simulink model "airTrackLab"  (R2021a)
settings: Solver=ode23t  StartTime=0.0  StopTime=30  FixedStep=0.02  MaxStep=0.01  RelTol=1e-3  AbsTol=1e-4  EnableMultiTasking=on
PostLoadFcn:
  | disp('default settings')
  | 
  | % Default starting positions
  | x0_cart1 = -0.2
  | x0_cart2 = 0.8
  | x0_gate1 = -0.4
  | x0_gate2 = 0.4
  | 
  | % How much damping the carts feel
  | dampingCoef = 0.01 % N/(m/s)
  | 
  | % Hanger damping
  | pulleyDamping = 0;
  | 
  | % Max measurement noise for the gates
  | noise_max = 0.01 % seconds
  | 
  | % How many time steps to show in the history
  | nHistory = 4
  | 
  | % Based on the provided STLs
  | cart_length = 0.15
  | 
  | subsystems = find_system(gcs,'BlockType','SubSystem');
  | p = Simulink.Mask.get(subsystems{1});
  | p.Parameters(1).Value = '-0.8';
  | p.Parameters(2).Value = '0';
  | p.Parameters(3).Value = '-0.4';
  | p.Parameters(4).Value = '0.4';
  | p.Parameters(5).Value = '0';
  | p.Parameters(6).Value = '0';
  | 
  | % Resize the model window
  | set(0,"Units","pixels")
  | sSize = get(0,"screensize");
  | set_param(gcs,'location',...
  |     [1,sSize(4)*0.01,round(sSize(3)/2),sSize(4)*0.96]);
  | 
  | % Reset the zoom
  | set_param(gcs, 'ZoomFactor','FitSystem')
undefined symbols (not defined in the file): X, Y, Z
libraries: sm_lib x104, simulink x12, nesl_utility x9
(part 3 of 3)

== system airTrackLab/Air track model/Mass Cart 1/Plates 3 ==
  Plate 1 : sm_lib/Body Elements/File Solid  ExtGeomFileName=weight.stl  UnitType=Custom  ExtGeomFileUnits=mm  StepReaderType=HEX  ExportConvexHullGeometry=off  InertiaType=PointMass  Mass=100  MassUnits=g  CenterOfMass=[0 0 0]  CenterOfMassUnits=m  MomentsOfInertia=[1 1 1]  MomentsOfInertiaUnits=kg*m^2  ProductsOfInertia=[0 0 0]  ProductsOfInertiaUnits=kg*m^2  BasedOnType=Density  Density=1000  DensityUnits=kg/m^3  DoExposeReferenceFrame=on  SerializedFrames=<Frames/>  GraphicType=FromGeometry  MarkerShape=Sphere  MarkerSize=10  GraphicVisPropType=AdvancedVisualProperties  GraphicDiffuseColor="[0.70   0.7    0.3]"  GraphicSpecularColor="[0.7  0.7  0.5 1]"  GraphicAmbientColor=[0.05 0.05 0.05 1]  GraphicEmissiveColor=[0.2 0.2 0.2 1.0]  GraphicShininess=3  GraphicOpacity=1.0
  Plate 2 : sm_lib/Body Elements/File Solid  ExtGeomFileName=weight.stl  UnitType=Custom  ExtGeomFileUnits=mm  StepReaderType=HEX  ExportConvexHullGeometry=off  InertiaType=PointMass  Mass=100  MassUnits=g  CenterOfMass=[0 0 0]  CenterOfMassUnits=m  MomentsOfInertia=[1 1 1]  MomentsOfInertiaUnits=kg*m^2  ProductsOfInertia=[0 0 0]  ProductsOfInertiaUnits=kg*m^2  BasedOnType=Density  Density=1000  DensityUnits=kg/m^3  DoExposeReferenceFrame=on  SerializedFrames=<Frames/>  GraphicType=FromGeometry  MarkerShape=Sphere  MarkerSize=10  GraphicVisPropType=AdvancedVisualProperties  GraphicDiffuseColor="[0.70   0.7    0.3]"  GraphicSpecularColor="[0.7  0.7  0.5 1]"  GraphicAmbientColor=[0.05 0.05 0.05 1]  GraphicEmissiveColor=[0.2 0.2 0.2 1.0]  GraphicShininess=3  GraphicOpacity=1.0
  Plate 3 : sm_lib/Body Elements/File Solid  ExtGeomFileName=weight.stl  UnitType=Custom  ExtGeomFileUnits=mm  StepReaderType=HEX  ExportConvexHullGeometry=off  InertiaType=PointMass  Mass=100  MassUnits=g  CenterOfMass=[0 0 0]  CenterOfMassUnits=m  MomentsOfInertia=[1 1 1]  MomentsOfInertiaUnits=kg*m^2  ProductsOfInertia=[0 0 0]  ProductsOfInertiaUnits=kg*m^2  BasedOnType=Density  Density=1000  DensityUnits=kg/m^3  DoExposeReferenceFrame=on  SerializedFrames=<Frames/>  GraphicType=FromGeometry  MarkerShape=Sphere  MarkerSize=10  GraphicVisPropType=AdvancedVisualProperties  GraphicDiffuseColor="[0.70   0.7    0.3]"  GraphicSpecularColor="[0.7  0.7  0.5 1]"  GraphicAmbientColor=[0.05 0.05 0.05 1]  GraphicEmissiveColor=[0.2 0.2 0.2 1.0]  GraphicShininess=3  GraphicOpacity=1.0
  Transform Plate 1 : sm_lib/Frames and Transforms/Rigid Transform  TranslationMethod=Cartesian  TranslationStandardOffset=0  TranslationLengthUnit=m  TranslationStandardAxis=+Z  TranslationCartesianOffset=[0 0.0055 0.0]  TranslationROffset=0  TranslationROffsetUnits=m  TranslationZOffset=0  TranslationZOffsetUnits=m  TranslationThetaOffset=0  TranslationThetaOffsetUnits=deg  RotationMethod=None  RotationAngleUnits=deg  RotationStandardAxis=+Z  RotationAngle=0.0  RotationArbitraryAxis=[0 0 1]  FollAlignAxisA=+X  BaseAlignAxisA=+Y  FollAlignAxisB=+Y  BaseAlignAxisB=+Z  RotationSequenceAxes=FollowerAxes  RotationSequence=XYX  RotationSequenceAngles=[0 0 0]  RotationSequenceAnglesUnits=deg  RotationMatrix=[1 0 0; 0 1 0; 0 0 1]
  Transform Plate 2 : sm_lib/Frames and Transforms/Rigid Transform  TranslationMethod=Cartesian  TranslationStandardOffset=0  TranslationLengthUnit=m  TranslationStandardAxis=+Z  TranslationCartesianOffset=[0 0.0055 0.0]  TranslationROffset=0  TranslationROffsetUnits=m  TranslationZOffset=0  TranslationZOffsetUnits=m  TranslationThetaOffset=0  TranslationThetaOffsetUnits=deg  RotationMethod=None  RotationAngleUnits=deg  RotationStandardAxis=+Z  RotationAngle=0.0  RotationArbitraryAxis=[0 0 1]  FollAlignAxisA=+X  BaseAlignAxisA=+Y  FollAlignAxisB=+Y  BaseAlignAxisB=+Z  RotationSequenceAxes=FollowerAxes  RotationSequence=XYX  RotationSequenceAngles=[0 0 0]  RotationSequenceAnglesUnits=deg  RotationMatrix=[1 0 0; 0 1 0; 0 0 1]
  Transform Plate 3 : sm_lib/Frames and Transforms/Rigid Transform  TranslationMethod=Cartesian  TranslationStandardOffset=0  TranslationLengthUnit=m  TranslationStandardAxis=+Z  TranslationCartesianOffset=[0 0.0055 0.0]  TranslationROffset=0  TranslationROffsetUnits=m  TranslationZOffset=0  TranslationZOffsetUnits=m  TranslationThetaOffset=0  TranslationThetaOffsetUnits=deg  RotationMethod=None  RotationAngleUnits=deg  RotationStandardAxis=+Z  RotationAngle=0.0  RotationArbitraryAxis=[0 0 1]  FollAlignAxisA=+X  BaseAlignAxisA=+Y  FollAlignAxisB=+Y  BaseAlignAxisB=+Z  RotationSequenceAxes=FollowerAxes  RotationSequence=XYX  RotationSequenceAngles=[0 0 0]  RotationSequenceAnglesUnits=deg  RotationMatrix=[1 0 0; 0 1 0; 0 0 1]
  B : PMIOPort  Side=Right
  connections:
  Plate 2/RConn1 -- Transform Plate 2/RConn1 -- Transform Plate 3/LConn1
  Transform Plate 1/LConn1 -- B/RConn1
  Transform Plate 2/LConn1 -- Plate 1/RConn1 -- Transform Plate 1/RConn1
  Plate 3/RConn1 -- Transform Plate 3/RConn1

== system airTrackLab/Air track model/Mass Cart 2/None  ==
  Reference Frame : sm_lib/Frames and Transforms/Reference Frame
  B : PMIOPort  Side=Right
  connections:
  B/RConn1 -- Reference Frame/RConn1

== system airTrackLab/Air track model/Mass Cart 2/Plates 1 ==
  Plate 1 : sm_lib/Body Elements/File Solid  ExtGeomFileName=weight.stl  UnitType=Custom  ExtGeomFileUnits=mm  StepReaderType=HEX  ExportConvexHullGeometry=off  InertiaType=PointMass  Mass=100  MassUnits=g  CenterOfMass=[0 0 0]  CenterOfMassUnits=m  MomentsOfInertia=[1 1 1]  MomentsOfInertiaUnits=kg*m^2  ProductsOfInertia=[0 0 0]  ProductsOfInertiaUnits=kg*m^2  BasedOnType=Density  Density=1000  DensityUnits=kg/m^3  DoExposeReferenceFrame=on  SerializedFrames=<Frames/>  GraphicType=FromGeometry  MarkerShape=Sphere  MarkerSize=10  GraphicVisPropType=AdvancedVisualProperties  GraphicDiffuseColor="[0.70   0.7    0.3]"  GraphicSpecularColor="[0.7  0.7  0.5 1]"  GraphicAmbientColor=[0.05 0.05 0.05 1]  GraphicEmissiveColor=[0.2 0.2 0.2 1.0]  GraphicShininess=3  GraphicOpacity=1.0
  Transform Plate 1 : sm_lib/Frames and Transforms/Rigid Transform  TranslationMethod=Cartesian  TranslationStandardOffset=0  TranslationLengthUnit=m  TranslationStandardAxis=+Z  TranslationCartesianOffset=[0 0.0055 0.0]  TranslationROffset=0  TranslationROffsetUnits=m  TranslationZOffset=0  TranslationZOffsetUnits=m  TranslationThetaOffset=0  TranslationThetaOffsetUnits=deg  RotationMethod=None  RotationAngleUnits=deg  RotationStandardAxis=+Z  RotationAngle=0.0  RotationArbitraryAxis=[0 0 1]  FollAlignAxisA=+X  BaseAlignAxisA=+Y  FollAlignAxisB=+Y  BaseAlignAxisB=+Z  RotationSequenceAxes=FollowerAxes  RotationSequence=XYX  RotationSequenceAngles=[0 0 0]  RotationSequenceAnglesUnits=deg  RotationMatrix=[1 0 0; 0 1 0; 0 0 1]
  B : PMIOPort  Side=Right
  connections:
  Plate 1/RConn1 -- Transform Plate 1/RConn1
  Transform Plate 1/LConn1 -- B/RConn1

== system airTrackLab/Air track model/Mass Cart 2/Plates 2 ==
  Plate 1 : sm_lib/Body Elements/File Solid  ExtGeomFileName=weight.stl  UnitType=Custom  ExtGeomFileUnits=mm  StepReaderType=HEX  ExportConvexHullGeometry=off  InertiaType=PointMass  Mass=100  MassUnits=g  CenterOfMass=[0 0 0]  CenterOfMassUnits=m  MomentsOfInertia=[1 1 1]  MomentsOfInertiaUnits=kg*m^2  ProductsOfInertia=[0 0 0]  ProductsOfInertiaUnits=kg*m^2  BasedOnType=Density  Density=1000  DensityUnits=kg/m^3  DoExposeReferenceFrame=on  SerializedFrames=<Frames/>  GraphicType=FromGeometry  MarkerShape=Sphere  MarkerSize=10  GraphicVisPropType=AdvancedVisualProperties  GraphicDiffuseColor="[0.70   0.7    0.3]"  GraphicSpecularColor="[0.7  0.7  0.5 1]"  GraphicAmbientColor=[0.05 0.05 0.05 1]  GraphicEmissiveColor=[0.2 0.2 0.2 1.0]  GraphicShininess=3  GraphicOpacity=1.0
  Plate 2 : sm_lib/Body Elements/File Solid  ExtGeomFileName=weight.stl  UnitType=Custom  ExtGeomFileUnits=mm  StepReaderType=HEX  ExportConvexHullGeometry=off  InertiaType=PointMass  Mass=100  MassUnits=g  CenterOfMass=[0 0 0]  CenterOfMassUnits=m  MomentsOfInertia=[1 1 1]  MomentsOfInertiaUnits=kg*m^2  ProductsOfInertia=[0 0 0]  ProductsOfInertiaUnits=kg*m^2  BasedOnType=Density  Density=1000  DensityUnits=kg/m^3  DoExposeReferenceFrame=on  SerializedFrames=<Frames/>  GraphicType=FromGeometry  MarkerShape=Sphere  MarkerSize=10  GraphicVisPropType=AdvancedVisualProperties  GraphicDiffuseColor="[0.70   0.7    0.3]"  GraphicSpecularColor="[0.7  0.7  0.5 1]"  GraphicAmbientColor=[0.05 0.05 0.05 1]  GraphicEmissiveColor=[0.2 0.2 0.2 1.0]  GraphicShininess=3  GraphicOpacity=1.0
  Transform Plate 1 : sm_lib/Frames and Transforms/Rigid Transform  TranslationMethod=Cartesian  TranslationStandardOffset=0  TranslationLengthUnit=m  TranslationStandardAxis=+Z  TranslationCartesianOffset=[0 0.0055 0.0]  TranslationROffset=0  TranslationROffsetUnits=m  TranslationZOffset=0  TranslationZOffsetUnits=m  TranslationThetaOffset=0  TranslationThetaOffsetUnits=deg  RotationMethod=None  RotationAngleUnits=deg  RotationStandardAxis=+Z  RotationAngle=0.0  RotationArbitraryAxis=[0 0 1]  FollAlignAxisA=+X  BaseAlignAxisA=+Y  FollAlignAxisB=+Y  BaseAlignAxisB=+Z  RotationSequenceAxes=FollowerAxes  RotationSequence=XYX  RotationSequenceAngles=[0 0 0]  RotationSequenceAnglesUnits=deg  RotationMatrix=[1 0 0; 0 1 0; 0 0 1]
  Transform Plate 2 : sm_lib/Frames and Transforms/Rigid Transform  TranslationMethod=Cartesian  TranslationStandardOffset=0  TranslationLengthUnit=m  TranslationStandardAxis=+Z  TranslationCartesianOffset=[0 0.0055 0.0]  TranslationROffset=0  TranslationROffsetUnits=m  TranslationZOffset=0  TranslationZOffsetUnits=m  TranslationThetaOffset=0  TranslationThetaOffsetUnits=deg  RotationMethod=None  RotationAngleUnits=deg  RotationStandardAxis=+Z  RotationAngle=0.0  RotationArbitraryAxis=[0 0 1]  FollAlignAxisA=+X  BaseAlignAxisA=+Y  FollAlignAxisB=+Y  BaseAlignAxisB=+Z  RotationSequenceAxes=FollowerAxes  RotationSequence=XYX  RotationSequenceAngles=[0 0 0]  RotationSequenceAnglesUnits=deg  RotationMatrix=[1 0 0; 0 1 0; 0 0 1]
  B : PMIOPort  Side=Right
  connections:
  Plate 2/RConn1 -- Transform Plate 2/RConn1
  Transform Plate 1/LConn1 -- B/RConn1
  Transform Plate 1/RConn1 -- Transform Plate 2/LConn1 -- Plate 1/RConn1

== system airTrackLab/Air track model/Mass Cart 2/Plates 3 ==
  Plate 1 : sm_lib/Body Elements/File Solid  ExtGeomFileName=weight.stl  UnitType=Custom  ExtGeomFileUnits=mm  StepReaderType=HEX  ExportConvexHullGeometry=off  InertiaType=PointMass  Mass=100  MassUnits=g  CenterOfMass=[0 0 0]  CenterOfMassUnits=m  MomentsOfInertia=[1 1 1]  MomentsOfInertiaUnits=kg*m^2  ProductsOfInertia=[0 0 0]  ProductsOfInertiaUnits=kg*m^2  BasedOnType=Density  Density=1000  DensityUnits=kg/m^3  DoExposeReferenceFrame=on  SerializedFrames=<Frames/>  GraphicType=FromGeometry  MarkerShape=Sphere  MarkerSize=10  GraphicVisPropType=AdvancedVisualProperties  GraphicDiffuseColor="[0.70   0.7    0.3]"  GraphicSpecularColor="[0.7  0.7  0.5 1]"  GraphicAmbientColor=[0.05 0.05 0.05 1]  GraphicEmissiveColor=[0.2 0.2 0.2 1.0]  GraphicShininess=3  GraphicOpacity=1.0
  Plate 2 : sm_lib/Body Elements/File Solid  ExtGeomFileName=weight.stl  UnitType=Custom  ExtGeomFileUnits=mm  StepReaderType=HEX  ExportConvexHullGeometry=off  InertiaType=PointMass  Mass=100  MassUnits=g  CenterOfMass=[0 0 0]  CenterOfMassUnits=m  MomentsOfInertia=[1 1 1]  MomentsOfInertiaUnits=kg*m^2  ProductsOfInertia=[0 0 0]  ProductsOfInertiaUnits=kg*m^2  BasedOnType=Density  Density=1000  DensityUnits=kg/m^3  DoExposeReferenceFrame=on  SerializedFrames=<Frames/>  GraphicType=FromGeometry  MarkerShape=Sphere  MarkerSize=10  GraphicVisPropType=AdvancedVisualProperties  GraphicDiffuseColor="[0.70   0.7    0.3]"  GraphicSpecularColor="[0.7  0.7  0.5 1]"  GraphicAmbientColor=[0.05 0.05 0.05 1]  GraphicEmissiveColor=[0.2 0.2 0.2 1.0]  GraphicShininess=3  GraphicOpacity=1.0
  Plate 3 : sm_lib/Body Elements/File Solid  ExtGeomFileName=weight.stl  UnitType=Custom  ExtGeomFileUnits=mm  StepReaderType=HEX  ExportConvexHullGeometry=off  InertiaType=PointMass  Mass=100  MassUnits=g  CenterOfMass=[0 0 0]  CenterOfMassUnits=m  MomentsOfInertia=[1 1 1]  MomentsOfInertiaUnits=kg*m^2  ProductsOfInertia=[0 0 0]  ProductsOfInertiaUnits=kg*m^2  BasedOnType=Density  Density=1000  DensityUnits=kg/m^3  DoExposeReferenceFrame=on  SerializedFrames=<Frames/>  GraphicType=FromGeometry  MarkerShape=Sphere  MarkerSize=10  GraphicVisPropType=AdvancedVisualProperties  GraphicDiffuseColor="[0.70   0.7    0.3]"  GraphicSpecularColor="[0.7  0.7  0.5 1]"  GraphicAmbientColor=[0.05 0.05 0.05 1]  GraphicEmissiveColor=[0.2 0.2 0.2 1.0]  GraphicShininess=3  GraphicOpacity=1.0
  Transform Plate 1 : sm_lib/Frames and Transforms/Rigid Transform  TranslationMethod=Cartesian  TranslationStandardOffset=0  TranslationLengthUnit=m  TranslationStandardAxis=+Z  TranslationCartesianOffset=[0 0.0055 0.0]  TranslationROffset=0  TranslationROffsetUnits=m  TranslationZOffset=0  TranslationZOffsetUnits=m  TranslationThetaOffset=0  TranslationThetaOffsetUnits=deg  RotationMethod=None  RotationAngleUnits=deg  RotationStandardAxis=+Z  RotationAngle=0.0  RotationArbitraryAxis=[0 0 1]  FollAlignAxisA=+X  BaseAlignAxisA=+Y  FollAlignAxisB=+Y  BaseAlignAxisB=+Z  RotationSequenceAxes=FollowerAxes  RotationSequence=XYX  RotationSequenceAngles=[0 0 0]  RotationSequenceAnglesUnits=deg  RotationMatrix=[1 0 0; 0 1 0; 0 0 1]
  Transform Plate 2 : sm_lib/Frames and Transforms/Rigid Transform  TranslationMethod=Cartesian  TranslationStandardOffset=0  TranslationLengthUnit=m  TranslationStandardAxis=+Z  TranslationCartesianOffset=[0 0.0055 0.0]  TranslationROffset=0  TranslationROffsetUnits=m  TranslationZOffset=0  TranslationZOffsetUnits=m  TranslationThetaOffset=0  TranslationThetaOffsetUnits=deg  RotationMethod=None  RotationAngleUnits=deg  RotationStandardAxis=+Z  RotationAngle=0.0  RotationArbitraryAxis=[0 0 1]  FollAlignAxisA=+X  BaseAlignAxisA=+Y  FollAlignAxisB=+Y  BaseAlignAxisB=+Z  RotationSequenceAxes=FollowerAxes  RotationSequence=XYX  RotationSequenceAngles=[0 0 0]  RotationSequenceAnglesUnits=deg  RotationMatrix=[1 0 0; 0 1 0; 0 0 1]
  Transform Plate 3 : sm_lib/Frames and Transforms/Rigid Transform  TranslationMethod=Cartesian  TranslationStandardOffset=0  TranslationLengthUnit=m  TranslationStandardAxis=+Z  TranslationCartesianOffset=[0 0.0055 0.0]  TranslationROffset=0  TranslationROffsetUnits=m  TranslationZOffset=0  TranslationZOffsetUnits=m  TranslationThetaOffset=0  TranslationThetaOffsetUnits=deg  RotationMethod=None  RotationAngleUnits=deg  RotationStandardAxis=+Z  RotationAngle=0.0  RotationArbitraryAxis=[0 0 1]  FollAlignAxisA=+X  BaseAlignAxisA=+Y  FollAlignAxisB=+Y  BaseAlignAxisB=+Z  RotationSequenceAxes=FollowerAxes  RotationSequence=XYX  RotationSequenceAngles=[0 0 0]  RotationSequenceAnglesUnits=deg  RotationMatrix=[1 0 0; 0 1 0; 0 0 1]
  B : PMIOPort  Side=Right
  connections:
  Plate 3/RConn1 -- Transform Plate 3/RConn1
  Transform Plate 1/RConn1 -- Plate 1/RConn1 -- Transform Plate 2/LConn1
  Transform Plate 1/LConn1 -- B/RConn1
  Transform Plate 3/LConn1 -- Transform Plate 2/RConn1 -- Plate 2/RConn1

== system airTrackLab/Air track model/Force Cart 1/short pulse/Triggered Subsystem ==
  In1 : Inport
  Trigger : TriggerPort  VariantControl=Variant
  Out1 : Outport
  wires:
  In1/1 -> Out1/1

== system airTrackLab/Air track model/Force Cart 1/short pulse/Triggered Subsystem1 ==
  In1 : Inport
  Trigger : TriggerPort  VariantControl=Variant
  Out1 : Outport
  wires:
  In1/1 -> Out1/1

== system airTrackLab/Air track model/Force Cart 2/Interactive Pulse/Triggered Subsystem ==
  In1 : Inport
  Trigger : TriggerPort  VariantControl=Variant
  Out1 : Outport
  wires:
  In1/1 -> Out1/1

== system airTrackLab/Air track model/Force Cart 2/Interactive Pulse/Triggered Subsystem1 ==
  In1 : Inport
  Trigger : TriggerPort  VariantControl=Variant
  Out1 : Outport
  wires:
  In1/1 -> Out1/1

== system airTrackLab/Air track model/Gate 1/Gate timing and history/Gate Trigger1 ==
  note: If the cart passes close to the gate, take a recording
      | (only triggers once when it comes into range)
  position1 : Inport
  velocity1 : Inport  Port=2
  gate_pos : Inport  Port=3
  Abs : Abs
  Compare To Constant : simulink/Logic and Bit Operations/Compare To Constant  relop=<=  const=0.01  OutDataTypeStr=boolean
  Subtract : Sum  Inputs=+-
  Uniform Random Number1 : UniformRandomNumber  Minimum=-noise_max/2  Maximum=noise_max/2  SampleTime=0.1
  gate 1 recording : Subsystem  TreatAsAtomicUnit=on
  cart time : Outport
  wires:
  position1/1 -> Subtract/2
  velocity1/1 -> gate 1 recording/1(In1)
  gate 1 recording/1(cart time) -> cart time/1
  Abs/1 -> Compare To Constant/1
  Subtract/1 -> Abs/1
  Compare To Constant/1 -> gate 1 recording/Trigger
  Uniform Random Number1/1 -> gate 1 recording/2(In2)
  gate_pos/1 -> Subtract/1

== system airTrackLab/Air track model/Gate 1/Gate timing and history/Gate Trigger2 ==
  note: If the cart passes close to the gate, take a recording
      | (only triggers once when it comes into range)
  position1 : Inport
  velocity1 : Inport  Port=2
  gate_pos : Inport  Port=3
  Abs : Abs
  Compare To Constant : simulink/Logic and Bit Operations/Compare To Constant  relop=<=  const=0.01  OutDataTypeStr=boolean
  Subtract : Sum  Inputs=+-
  Uniform Random Number : UniformRandomNumber  Minimum=-noise_max/2  Maximum=noise_max/2  SampleTime=0.1
  gate 1 recording : Subsystem  TreatAsAtomicUnit=on
  cart time : Outport
  wires:
  position1/1 -> Subtract/2
  velocity1/1 -> gate 1 recording/1(In1)
  gate 1 recording/1(cart time) -> cart time/1
  Abs/1 -> Compare To Constant/1
  Subtract/1 -> Abs/1
  Compare To Constant/1 -> gate 1 recording/Trigger
  Uniform Random Number/1 -> gate 1 recording/2(In2)
  gate_pos/1 -> Subtract/1

== system airTrackLab/Air track model/Gate 1/Gate timing and history/Memory system ==
  value : Inport
  Assignment : Assignment  DiagnosticForDimensions=Warning  IndexOptions=Index vector (dialog)  Indices=1  OutputSizes=1
  Equal : RelationalOperator  Operator=~=  OutDataTypeStr=boolean  RndMeth=Simplest
  Triggered Subsystem : Subsystem  TreatAsAtomicUnit=on
  Unit Delay : UnitDelay  InitialCondition=zeros(nHistory,1)  SampleTime=-1  HasFrameUpgradeWarning=on
  Unit Delay1 : UnitDelay  SampleTime=-1  HasFrameUpgradeWarning=on
  last n values : Outport
  wires:
  Unit Delay/1 -> Triggered Subsystem/1(In1)
  Assignment/1 -> Unit Delay/1, last n values/1
  value/1 -> Equal/1, Unit Delay1/1, Assignment/2
  Triggered Subsystem/1(Out1) -> Assignment/1
  Equal/1 -> Triggered Subsystem/Trigger
  Unit Delay1/1 -> Equal/2

== system airTrackLab/Air track model/Gate 1/Gate timing and history/Triggered Subsystem ==
  time : Inport
  Trigger : TriggerPort  VariantControl=Variant
  timeOut : Outport
  wires:
  time/1 -> timeOut/1

== system airTrackLab/Air track model/Gate 2/Gate timing and history/Gate Trigger1 ==
  note: If the cart passes close to the gate, take a recording
      | (only triggers once when it comes into range)
  position1 : Inport
  velocity1 : Inport  Port=2
  gate_pos : Inport  Port=3
  Abs : Abs
  Compare To Constant : simulink/Logic and Bit Operations/Compare To Constant  relop=<=  const=0.01  OutDataTypeStr=boolean
  Subtract : Sum  Inputs=+-
  Uniform Random Number1 : UniformRandomNumber  Minimum=-noise_max/2  Maximum=noise_max/2  SampleTime=0.1
  gate 1 recording : Subsystem  TreatAsAtomicUnit=on
  cart time : Outport
  wires:
  position1/1 -> Subtract/2
  velocity1/1 -> gate 1 recording/1(In1)
  gate 1 recording/1(cart time) -> cart time/1
  Abs/1 -> Compare To Constant/1
  Subtract/1 -> Abs/1
  Compare To Constant/1 -> gate 1 recording/Trigger
  Uniform Random Number1/1 -> gate 1 recording/2(In2)
  gate_pos/1 -> Subtract/1

== system airTrackLab/Air track model/Gate 2/Gate timing and history/Gate Trigger2 ==
  note: If the cart passes close to the gate, take a recording
      | (only triggers once when it comes into range)
  position1 : Inport
  velocity1 : Inport  Port=2
  gate_pos : Inport  Port=3
  Abs : Abs
  Compare To Constant : simulink/Logic and Bit Operations/Compare To Constant  relop=<=  const=0.01  OutDataTypeStr=boolean
  Subtract : Sum  Inputs=+-
  Uniform Random Number1 : UniformRandomNumber  Minimum=-noise_max/2  Maximum=noise_max/2  SampleTime=0.1
  gate 1 recording : Subsystem  TreatAsAtomicUnit=on
  cart time : Outport
  wires:
  position1/1 -> Subtract/2
  velocity1/1 -> gate 1 recording/1(In1)
  gate 1 recording/1(cart time) -> cart time/1
  Abs/1 -> Compare To Constant/1
  Subtract/1 -> Abs/1
  Compare To Constant/1 -> gate 1 recording/Trigger
  Uniform Random Number1/1 -> gate 1 recording/2(In2)
  gate_pos/1 -> Subtract/1

== system airTrackLab/Air track model/Gate 2/Gate timing and history/Memory system ==
  value : Inport
  Assignment : Assignment  DiagnosticForDimensions=Warning  IndexOptions=Index vector (dialog)  Indices=1  OutputSizes=1
  Equal : RelationalOperator  Operator=~=  OutDataTypeStr=boolean  RndMeth=Simplest
  Triggered Subsystem : Subsystem  TreatAsAtomicUnit=on
  Unit Delay : UnitDelay  InitialCondition=zeros(nHistory,1)  SampleTime=-1  HasFrameUpgradeWarning=on
  Unit Delay1 : UnitDelay  SampleTime=-1  HasFrameUpgradeWarning=on
  last n values : Outport
  wires:
  Unit Delay/1 -> Triggered Subsystem/1(In1)
  Assignment/1 -> Unit Delay/1, last n values/1
  value/1 -> Equal/1, Unit Delay1/1, Assignment/2
  Triggered Subsystem/1(Out1) -> Assignment/1
  Equal/1 -> Triggered Subsystem/Trigger
  Unit Delay1/1 -> Equal/2

== system airTrackLab/Air track model/Gate 2/Gate timing and history/Triggered Subsystem ==
  time : Inport
  Trigger : TriggerPort  VariantControl=Variant
  timeOut : Outport
  wires:
  time/1 -> timeOut/1

== system airTrackLab/Air track model/Load/Hanging Mass/Hook ==
  Rigid Transform11 : sm_lib/Frames and Transforms/Rigid Transform  TranslationMethod=Cartesian  TranslationStandardOffset=1  TranslationLengthUnit=m  TranslationStandardAxis=+X  TranslationCartesianOffset=[1.045 -0.18 0]  TranslationROffset=0  TranslationROffsetUnits=m  TranslationZOffset=0  TranslationZOffsetUnits=m  TranslationThetaOffset=0  TranslationThetaOffsetUnits=deg  RotationMethod=None  RotationAngleUnits=deg  RotationStandardAxis=+Z  RotationAngle=0.0  RotationArbitraryAxis=[0 0 1]  FollAlignAxisA=+X  BaseAlignAxisA=+Y  FollAlignAxisB=+Y  BaseAlignAxisB=+Z  RotationSequenceAxes=FollowerAxes  RotationSequence=XYX  RotationSequenceAngles=[0 0 0]  RotationSequenceAnglesUnits=deg  RotationMatrix=[1 0 0; 0 1 0; 0 0 1]
  Rigid Transform13 : sm_lib/Frames and Transforms/Rigid Transform  TranslationMethod=Cartesian  TranslationStandardOffset=0.1  TranslationLengthUnit=m  TranslationStandardAxis=-Y  TranslationCartesianOffset=[0 0.313 0]  TranslationROffset=0  TranslationROffsetUnits=m  TranslationZOffset=0  TranslationZOffsetUnits=m  TranslationThetaOffset=0  TranslationThetaOffsetUnits=deg  RotationMethod=None  RotationAngleUnits=deg  RotationStandardAxis=-Y  RotationAngle=0.0  RotationArbitraryAxis=[0 0 1]  FollAlignAxisA=+X  BaseAlignAxisA=+Y  FollAlignAxisB=+Y  BaseAlignAxisB=+Z  RotationSequenceAxes=FollowerAxes  RotationSequence=XYX  RotationSequenceAngles=[0 0 0]  RotationSequenceAnglesUnits=deg  RotationMatrix=[1 0 0; 0 1 0; 0 0 1]
  mass hanger : sm_lib/Body Elements/File Solid  ExtGeomFileName=hanger.stl  UnitType=Custom  ExtGeomFileUnits=mm  StepReaderType=HEX  ExportConvexHullGeometry=off  InertiaType=PointMass  Mass=0  MassUnits=g  CenterOfMass=[0 0 0]  CenterOfMassUnits=m  MomentsOfInertia=[1 1 1]  MomentsOfInertiaUnits=kg*m^2  ProductsOfInertia=[0 0 0]  ProductsOfInertiaUnits=kg*m^2  BasedOnType=Density  Density=1000  DensityUnits=kg/m^3  DoExposeReferenceFrame=on  SerializedFrames=<Frames/>  GraphicType=FromGeometry  MarkerShape=Sphere  MarkerSize=10  GraphicVisPropType=AdvancedVisualProperties  GraphicDiffuseColor="[0.8   0.8    0.8]"  GraphicSpecularColor="[0.8    0.8   0.8 1]"  GraphicAmbientColor=[0.05 0.05 0.05 1]  GraphicEmissiveColor=[0.0 0.0 0.0 1.0]  GraphicShininess=5  GraphicOpacity=1.0
  M : PMIOPort  Side=Right
  C : PMIOPort  Port=2  Side=Left
  connections:
  Rigid Transform13/RConn1 -- C/RConn1 -- Rigid Transform11/LConn1
  M/RConn1 -- Rigid Transform13/LConn1
  mass hanger/RConn1 -- Rigid Transform11/RConn1

== system airTrackLab/Air track model/Load/Hanging Mass/Mass ==
  "None " : Subsystem  VariantControl=None
      mask Display: disp(' ');
  Plates 1 : Subsystem  VariantControl=Plates_1
      mask Display: image('Plates_1.png');
  Plates 2 : Subsystem  VariantControl=Plates_2
      mask Display: image('Plates_2.png');
  Plates 3 : Subsystem  VariantControl=Plates_3
      mask Display: image('Plates_3.png');
  B : PMIOPort  Side=Right

== system airTrackLab/Air track model/Load/Hanging Mass/Pulley ==
  Pulley : sm_lib/Body Elements/File Solid  ExtGeomFileName=wheel.stl  UnitType=Custom  ExtGeomFileUnits=mm  StepReaderType=HEX  ExportConvexHullGeometry=off  InertiaType=CalculateFromGeometry  Mass=180  MassUnits=g  CenterOfMass=[0 0 0]  CenterOfMassUnits=m  MomentsOfInertia=[1 1 1]  MomentsOfInertiaUnits=kg*m^2  ProductsOfInertia=[0 0 0]  ProductsOfInertiaUnits=kg*m^2  BasedOnType=Density  Density=1000  DensityUnits=kg/m^3  DoExposeReferenceFrame=off  SerializedFrames=<Frames><Frame><Id>Frame1</Id><Value><Name>F1</Name><Origin><Source>CenterOfMassFrame</Source><FeatureName></FeatureName></Origin><PrimaryAxis><DefinedDirection>+Z</DefinedDirection><Source>ReferenceFrame</Source><SourceDirection>+Z</SourceDirection><FeatureName></FeatureName></PrimaryAxis><SecondaryAxis><DefinedDirection>+Y</DefinedDirection><Source>ReferenceFrame</Source><SourceDirection>+Y</SourceDirection><FeatureName></FeatureName></SecondaryAxis></Value></Frame></Frames>  GraphicType=FromGeometry  MarkerShape=Sphere  MarkerSize=10  GraphicVisPropType=AdvancedVisualProperties  GraphicDiffuseColor="[0.8   0.8    0.8]"  GraphicSpecularColor="[0.8    0.8   0.8 1]"  GraphicAmbientColor=[0.05 0.05 0.05 1]  GraphicEmissiveColor=[0.0 0.0 0.0 1.0]  GraphicShininess=5  GraphicOpacity=1.0
  Pulley Constraint : sm_lib/Belts and Cables/Pulley  PitchRadius=0.0235  PitchRadiusUnits=m  InitialWrapAngleLowerBound=0  InitialWrapAngleLowerBoundUnits=deg  SenseWrapAngle=off  SensePulleyAngleA=off  SensePulleyAngleB=off  SenseFleetAngleA=off  SenseFleetAngleB=off
      settings: SourceProductBaseCode=MS
  R : PMIOPort  Side=Left
  A : PMIOPort  Port=2  Side=Right
  B : PMIOPort  Port=3  Side=Right
  connections:
  Pulley Constraint/RConn2 -- B/RConn1
  Pulley Constraint/LConn1 -- Pulley/LConn1 -- R/RConn1
  Pulley Constraint/RConn1 -- A/RConn1

== system airTrackLab/Air track model/Gate 1/Gate timing and history/Gate Trigger1/gate 1 recording ==
  In1 : Inport
  In2 : Inport  Port=2
  Trigger : TriggerPort  VariantControl=Variant
  Abs : Abs
  Divide : Product  Inputs=*/
  Sum : Sum  Inputs=|++
  cart length (meters) : Constant  Value=cart_length
  cart time : Outport
  wires:
  In2/1 -> Sum/2
  Sum/1 -> cart time/1
  Abs/1 -> Sum/1
  Divide/1 -> Abs/1
  In1/1 -> Divide/2
  cart length (meters)/1 -> Divide/1

== system airTrackLab/Air track model/Gate 1/Gate timing and history/Gate Trigger2/gate 1 recording ==
  In1 : Inport
  In2 : Inport  Port=2
  Trigger : TriggerPort  VariantControl=Variant
  Abs : Abs
  Divide : Product  Inputs=*/
  Sum : Sum  Inputs=|++
  cart length (meters) : Constant  Value=cart_length
  cart time : Outport
  wires:
  In2/1 -> Sum/2
  Sum/1 -> cart time/1
  Abs/1 -> Sum/1
  Divide/1 -> Abs/1
  In1/1 -> Divide/2
  cart length (meters)/1 -> Divide/1

== system airTrackLab/Air track model/Gate 1/Gate timing and history/Memory system/Triggered Subsystem ==
  In1 : Inport
  Trigger : TriggerPort  VariantControl=Variant
  For Iterator Subsystem : Subsystem  TreatAsAtomicUnit=on
  Out1 : Outport
  wires:
  In1/1 -> For Iterator Subsystem/1(In1)
  For Iterator Subsystem/1(Out1) -> Out1/1

== system airTrackLab/Air track model/Gate 2/Gate timing and history/Gate Trigger1/gate 1 recording ==
  In1 : Inport
  In2 : Inport  Port=2
  Trigger : TriggerPort  VariantControl=Variant
  Abs : Abs
  Divide : Product  Inputs=*/
  Sum : Sum  Inputs=|++
  cart length (meters) : Constant  Value=cart_length
  cart time : Outport
  wires:
  In2/1 -> Sum/2
  Sum/1 -> cart time/1
  Abs/1 -> Sum/1
  Divide/1 -> Abs/1
  In1/1 -> Divide/2
  cart length (meters)/1 -> Divide/1

== system airTrackLab/Air track model/Gate 2/Gate timing and history/Gate Trigger2/gate 1 recording ==
  In1 : Inport
  In2 : Inport  Port=2
  Trigger : TriggerPort  VariantControl=Variant
  Abs : Abs
  Divide : Product  Inputs=*/
  Sum : Sum  Inputs=|++
  cart length (meters) : Constant  Value=cart_length
  cart time : Outport
  wires:
  In2/1 -> Sum/2
  Sum/1 -> cart time/1
  Abs/1 -> Sum/1
  Divide/1 -> Abs/1
  In1/1 -> Divide/2
  cart length (meters)/1 -> Divide/1

== system airTrackLab/Air track model/Gate 2/Gate timing and history/Memory system/Triggered Subsystem ==
  In1 : Inport
  Trigger : TriggerPort  VariantControl=Variant
  For Iterator Subsystem : Subsystem  TreatAsAtomicUnit=on
  Out1 : Outport
  wires:
  In1/1 -> For Iterator Subsystem/1(In1)
  For Iterator Subsystem/1(Out1) -> Out1/1

== system airTrackLab/Air track model/Load/Hanging Mass/Mass/None  ==
  Reference Frame : sm_lib/Frames and Transforms/Reference Frame
  B : PMIOPort  Side=Right
  connections:
  B/RConn1 -- Reference Frame/RConn1

== system airTrackLab/Air track model/Load/Hanging Mass/Mass/Plates 1 ==
  Plate 1 : sm_lib/Body Elements/File Solid  ExtGeomFileName=weight.stl  UnitType=Custom  ExtGeomFileUnits=mm  StepReaderType=HEX  ExportConvexHullGeometry=off  InertiaType=PointMass  Mass=100  MassUnits=g  CenterOfMass=[0 0 0]  CenterOfMassUnits=m  MomentsOfInertia=[1 1 1]  MomentsOfInertiaUnits=kg*m^2  ProductsOfInertia=[0 0 0]  ProductsOfInertiaUnits=kg*m^2  BasedOnType=Density  Density=1000  DensityUnits=kg/m^3  DoExposeReferenceFrame=on  SerializedFrames=<Frames/>  GraphicType=FromGeometry  MarkerShape=Sphere  MarkerSize=10  GraphicVisPropType=AdvancedVisualProperties  GraphicDiffuseColor="[0.70   0.7    0.3]"  GraphicSpecularColor="[0.7  0.7  0.5 1]"  GraphicAmbientColor=[0.05 0.05 0.05 1]  GraphicEmissiveColor=[0.2 0.2 0.2 1.0]  GraphicShininess=3  GraphicOpacity=1.0
  Transform Plate 1 : sm_lib/Frames and Transforms/Rigid Transform  TranslationMethod=Cartesian  TranslationStandardOffset=0  TranslationLengthUnit=m  TranslationStandardAxis=+Z  TranslationCartesianOffset=[0 0.0055 0.0]  TranslationROffset=0  TranslationROffsetUnits=m  TranslationZOffset=0  TranslationZOffsetUnits=m  TranslationThetaOffset=0  TranslationThetaOffsetUnits=deg  RotationMethod=None  RotationAngleUnits=deg  RotationStandardAxis=+Z  RotationAngle=0.0  RotationArbitraryAxis=[0 0 1]  FollAlignAxisA=+X  BaseAlignAxisA=+Y  FollAlignAxisB=+Y  BaseAlignAxisB=+Z  RotationSequenceAxes=FollowerAxes  RotationSequence=XYX  RotationSequenceAngles=[0 0 0]  RotationSequenceAnglesUnits=deg  RotationMatrix=[1 0 0; 0 1 0; 0 0 1]
  B : PMIOPort  Side=Right
  connections:
  Plate 1/RConn1 -- Transform Plate 1/RConn1
  Transform Plate 1/LConn1 -- B/RConn1

== system airTrackLab/Air track model/Load/Hanging Mass/Mass/Plates 2 ==
  Plate 1 : sm_lib/Body Elements/File Solid  ExtGeomFileName=weight.stl  UnitType=Custom  ExtGeomFileUnits=mm  StepReaderType=HEX  ExportConvexHullGeometry=off  InertiaType=PointMass  Mass=100  MassUnits=g  CenterOfMass=[0 0 0]  CenterOfMassUnits=m  MomentsOfInertia=[1 1 1]  MomentsOfInertiaUnits=kg*m^2  ProductsOfInertia=[0 0 0]  ProductsOfInertiaUnits=kg*m^2  BasedOnType=Density  Density=1000  DensityUnits=kg/m^3  DoExposeReferenceFrame=on  SerializedFrames=<Frames/>  GraphicType=FromGeometry  MarkerShape=Sphere  MarkerSize=10  GraphicVisPropType=AdvancedVisualProperties  GraphicDiffuseColor="[0.70   0.7    0.3]"  GraphicSpecularColor="[0.7  0.7  0.5 1]"  GraphicAmbientColor=[0.05 0.05 0.05 1]  GraphicEmissiveColor=[0.2 0.2 0.2 1.0]  GraphicShininess=3  GraphicOpacity=1.0
  Plate 2 : sm_lib/Body Elements/File Solid  ExtGeomFileName=weight.stl  UnitType=Custom  ExtGeomFileUnits=mm  StepReaderType=HEX  ExportConvexHullGeometry=off  InertiaType=PointMass  Mass=100  MassUnits=g  CenterOfMass=[0 0 0]  CenterOfMassUnits=m  MomentsOfInertia=[1 1 1]  MomentsOfInertiaUnits=kg*m^2  ProductsOfInertia=[0 0 0]  ProductsOfInertiaUnits=kg*m^2  BasedOnType=Density  Density=1000  DensityUnits=kg/m^3  DoExposeReferenceFrame=on  SerializedFrames=<Frames/>  GraphicType=FromGeometry  MarkerShape=Sphere  MarkerSize=10  GraphicVisPropType=AdvancedVisualProperties  GraphicDiffuseColor="[0.70   0.7    0.3]"  GraphicSpecularColor="[0.7  0.7  0.5 1]"  GraphicAmbientColor=[0.05 0.05 0.05 1]  GraphicEmissiveColor=[0.2 0.2 0.2 1.0]  GraphicShininess=3  GraphicOpacity=1.0
  Transform Plate 1 : sm_lib/Frames and Transforms/Rigid Transform  TranslationMethod=Cartesian  TranslationStandardOffset=0  TranslationLengthUnit=m  TranslationStandardAxis=+Z  TranslationCartesianOffset=[0 0.0055 0.0]  TranslationROffset=0  TranslationROffsetUnits=m  TranslationZOffset=0  TranslationZOffsetUnits=m  TranslationThetaOffset=0  TranslationThetaOffsetUnits=deg  RotationMethod=None  RotationAngleUnits=deg  RotationStandardAxis=+Z  RotationAngle=0.0  RotationArbitraryAxis=[0 0 1]  FollAlignAxisA=+X  BaseAlignAxisA=+Y  FollAlignAxisB=+Y  BaseAlignAxisB=+Z  RotationSequenceAxes=FollowerAxes  RotationSequence=XYX  RotationSequenceAngles=[0 0 0]  RotationSequenceAnglesUnits=deg  RotationMatrix=[1 0 0; 0 1 0; 0 0 1]
  Transform Plate 2 : sm_lib/Frames and Transforms/Rigid Transform  TranslationMethod=Cartesian  TranslationStandardOffset=0  TranslationLengthUnit=m  TranslationStandardAxis=+Z  TranslationCartesianOffset=[0 0.0055 0.0]  TranslationROffset=0  TranslationROffsetUnits=m  TranslationZOffset=0  TranslationZOffsetUnits=m  TranslationThetaOffset=0  TranslationThetaOffsetUnits=deg  RotationMethod=None  RotationAngleUnits=deg  RotationStandardAxis=+Z  RotationAngle=0.0  RotationArbitraryAxis=[0 0 1]  FollAlignAxisA=+X  BaseAlignAxisA=+Y  FollAlignAxisB=+Y  BaseAlignAxisB=+Z  RotationSequenceAxes=FollowerAxes  RotationSequence=XYX  RotationSequenceAngles=[0 0 0]  RotationSequenceAnglesUnits=deg  RotationMatrix=[1 0 0; 0 1 0; 0 0 1]
  B : PMIOPort  Side=Right
  connections:
  Plate 2/RConn1 -- Transform Plate 2/RConn1
  Transform Plate 1/LConn1 -- B/RConn1
  Transform Plate 1/RConn1 -- Transform Plate 2/LConn1 -- Plate 1/RConn1

== system airTrackLab/Air track model/Load/Hanging Mass/Mass/Plates 3 ==
  Plate 1 : sm_lib/Body Elements/File Solid  ExtGeomFileName=weight.stl  UnitType=Custom  ExtGeomFileUnits=mm  StepReaderType=HEX  ExportConvexHullGeometry=off  InertiaType=PointMass  Mass=100  MassUnits=g  CenterOfMass=[0 0 0]  CenterOfMassUnits=m  MomentsOfInertia=[1 1 1]  MomentsOfInertiaUnits=kg*m^2  ProductsOfInertia=[0 0 0]  ProductsOfInertiaUnits=kg*m^2  BasedOnType=Density  Density=1000  DensityUnits=kg/m^3  DoExposeReferenceFrame=on  SerializedFrames=<Frames/>  GraphicType=FromGeometry  MarkerShape=Sphere  MarkerSize=10  GraphicVisPropType=AdvancedVisualProperties  GraphicDiffuseColor="[0.70   0.7    0.3]"  GraphicSpecularColor="[0.7  0.7  0.5 1]"  GraphicAmbientColor=[0.05 0.05 0.05 1]  GraphicEmissiveColor=[0.2 0.2 0.2 1.0]  GraphicShininess=3  GraphicOpacity=1.0
  Plate 2 : sm_lib/Body Elements/File Solid  ExtGeomFileName=weight.stl  UnitType=Custom  ExtGeomFileUnits=mm  StepReaderType=HEX  ExportConvexHullGeometry=off  InertiaType=PointMass  Mass=100  MassUnits=g  CenterOfMass=[0 0 0]  CenterOfMassUnits=m  MomentsOfInertia=[1 1 1]  MomentsOfInertiaUnits=kg*m^2  ProductsOfInertia=[0 0 0]  ProductsOfInertiaUnits=kg*m^2  BasedOnType=Density  Density=1000  DensityUnits=kg/m^3  DoExposeReferenceFrame=on  SerializedFrames=<Frames/>  GraphicType=FromGeometry  MarkerShape=Sphere  MarkerSize=10  GraphicVisPropType=AdvancedVisualProperties  GraphicDiffuseColor="[0.70   0.7    0.3]"  GraphicSpecularColor="[0.7  0.7  0.5 1]"  GraphicAmbientColor=[0.05 0.05 0.05 1]  GraphicEmissiveColor=[0.2 0.2 0.2 1.0]  GraphicShininess=3  GraphicOpacity=1.0
  Plate 3 : sm_lib/Body Elements/File Solid  ExtGeomFileName=weight.stl  UnitType=Custom  ExtGeomFileUnits=mm  StepReaderType=HEX  ExportConvexHullGeometry=off  InertiaType=PointMass  Mass=100  MassUnits=g  CenterOfMass=[0 0 0]  CenterOfMassUnits=m  MomentsOfInertia=[1 1 1]  MomentsOfInertiaUnits=kg*m^2  ProductsOfInertia=[0 0 0]  ProductsOfInertiaUnits=kg*m^2  BasedOnType=Density  Density=1000  DensityUnits=kg/m^3  DoExposeReferenceFrame=on  SerializedFrames=<Frames/>  GraphicType=FromGeometry  MarkerShape=Sphere  MarkerSize=10  GraphicVisPropType=AdvancedVisualProperties  GraphicDiffuseColor="[0.70   0.7    0.3]"  GraphicSpecularColor="[0.7  0.7  0.5 1]"  GraphicAmbientColor=[0.05 0.05 0.05 1]  GraphicEmissiveColor=[0.2 0.2 0.2 1.0]  GraphicShininess=3  GraphicOpacity=1.0
  Transform Plate 1 : sm_lib/Frames and Transforms/Rigid Transform  TranslationMethod=Cartesian  TranslationStandardOffset=0  TranslationLengthUnit=m  TranslationStandardAxis=+Z  TranslationCartesianOffset=[0 0.0055 0.0]  TranslationROffset=0  TranslationROffsetUnits=m  TranslationZOffset=0  TranslationZOffsetUnits=m  TranslationThetaOffset=0  TranslationThetaOffsetUnits=deg  RotationMethod=None  RotationAngleUnits=deg  RotationStandardAxis=+Z  RotationAngle=0.0  RotationArbitraryAxis=[0 0 1]  FollAlignAxisA=+X  BaseAlignAxisA=+Y  FollAlignAxisB=+Y  BaseAlignAxisB=+Z  RotationSequenceAxes=FollowerAxes  RotationSequence=XYX  RotationSequenceAngles=[0 0 0]  RotationSequenceAnglesUnits=deg  RotationMatrix=[1 0 0; 0 1 0; 0 0 1]
  Transform Plate 2 : sm_lib/Frames and Transforms/Rigid Transform  TranslationMethod=Cartesian  TranslationStandardOffset=0  TranslationLengthUnit=m  TranslationStandardAxis=+Z  TranslationCartesianOffset=[0 0.0055 0.0]  TranslationROffset=0  TranslationROffsetUnits=m  TranslationZOffset=0  TranslationZOffsetUnits=m  TranslationThetaOffset=0  TranslationThetaOffsetUnits=deg  RotationMethod=None  RotationAngleUnits=deg  RotationStandardAxis=+Z  RotationAngle=0.0  RotationArbitraryAxis=[0 0 1]  FollAlignAxisA=+X  BaseAlignAxisA=+Y  FollAlignAxisB=+Y  BaseAlignAxisB=+Z  RotationSequenceAxes=FollowerAxes  RotationSequence=XYX  RotationSequenceAngles=[0 0 0]  RotationSequenceAnglesUnits=deg  RotationMatrix=[1 0 0; 0 1 0; 0 0 1]
  Transform Plate 3 : sm_lib/Frames and Transforms/Rigid Transform  TranslationMethod=Cartesian  TranslationStandardOffset=0  TranslationLengthUnit=m  TranslationStandardAxis=+Z  TranslationCartesianOffset=[0 0.0055 0.0]  TranslationROffset=0  TranslationROffsetUnits=m  TranslationZOffset=0  TranslationZOffsetUnits=m  TranslationThetaOffset=0  TranslationThetaOffsetUnits=deg  RotationMethod=None  RotationAngleUnits=deg  RotationStandardAxis=+Z  RotationAngle=0.0  RotationArbitraryAxis=[0 0 1]  FollAlignAxisA=+X  BaseAlignAxisA=+Y  FollAlignAxisB=+Y  BaseAlignAxisB=+Z  RotationSequenceAxes=FollowerAxes  RotationSequence=XYX  RotationSequenceAngles=[0 0 0]  RotationSequenceAnglesUnits=deg  RotationMatrix=[1 0 0; 0 1 0; 0 0 1]
  B : PMIOPort  Side=Right
  connections:
  Plate 3/RConn1 -- Transform Plate 3/RConn1
  Plate 1/RConn1 -- Transform Plate 1/RConn1 -- Transform Plate 2/LConn1
  Transform Plate 1/LConn1 -- B/RConn1
  Transform Plate 2/RConn1 -- Plate 2/RConn1 -- Transform Plate 3/LConn1

== system airTrackLab/Air track model/Gate 1/Gate timing and history/Memory system/Triggered Subsystem/For Iterator Subsystem ==
  In1 : Inport
  Assignment : Assignment  DiagnosticForDimensions=Warning  IndexOptions=Index vector (port)  Indices=1  OutputSizes=1
  Bias : Bias  Bias=1
  For Iterator : ForIterator  IterationLimit=nHistory-1
  Selector : Selector  InputPortWidth=nHistory  IndexOptions=Index vector (port)  Indices=[1 3]  OutputSizes=1
  Out1 : Outport
  wires:
  For Iterator/1 -> Bias/1, Selector/2
  Assignment/1 -> Out1/1
  In1/1 -> Assignment/1, Selector/1
  Bias/1 -> Assignment/3
  Selector/1 -> Assignment/2

== system airTrackLab/Air track model/Gate 2/Gate timing and history/Memory system/Triggered Subsystem/For Iterator Subsystem ==
  In1 : Inport
  Assignment : Assignment  DiagnosticForDimensions=Warning  IndexOptions=Index vector (port)  Indices=1  OutputSizes=1
  Bias : Bias  Bias=1
  For Iterator : ForIterator  IterationLimit=nHistory-1
  Selector : Selector  InputPortWidth=nHistory  IndexOptions=Index vector (port)  Indices=[1 3]  OutputSizes=1
  Out1 : Outport
  wires:
  For Iterator/1 -> Bias/1, Selector/2
  Assignment/1 -> Out1/1
  In1/1 -> Assignment/1, Selector/1
  Bias/1 -> Assignment/3
  Selector/1 -> Assignment/2
